simulink model "Versie1"  (Simulink 7.9)
settings: Solver=ode15s  StartTime=0.0  StopTime=10*24*3600  RelTol=1e-3
undefined symbols (not defined in the file or in its folder): B, U, x0
settings Model: Creator=psross  LastModifiedBy=M.Sparnaaij  ExtModeTrigMode=oneshot  ExtModeArmWhenConnect=off
settings DataIOCC: LimitDataPoints=off  SignalLoggingName=sigsOut
settings OptimizationCC: BooleanDataType=off
settings DebuggingCC: SaveWithParameterizedLinksMsg=none  SignalResolutionControl=TryResolveAllWithWarning  SolverPrmCheckMsg=none  MultiTaskDSMMsg=warning  MultiTaskCondExecSysMsg=none  StrictBusMsg=None
settings HardwareCC: TargetUnknown=on
settings RTWCC: IncludeERTFirstTime=on
settings GRTTargetCC: TargetFcnLib=ansi_tfl_tmw.mat  CombineOutputUpdateFcns=off  GRTInterface=on

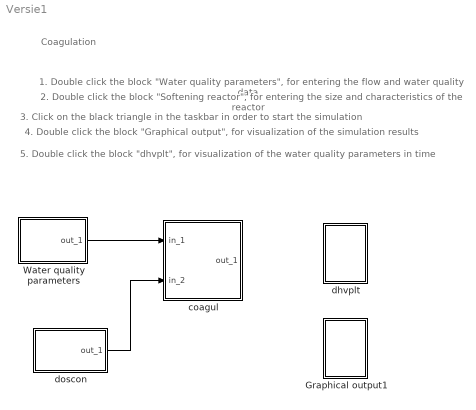
== system Versie1 ==
  note: Coagulation
  note: 3. Click on the black triangle in the taskbar in order to start the simulation
  note: 4. Double click the block "Graphical output", for visualization of the simulation results
  note: 1. Double click the block "Water quality parameters", for entering the flow and water quality data
  note: 2. Double click the block "Softening reactor", for entering the size and characteristics of the reactor
  note: 5. Double click the block "dhvplt", for visualization of the water quality parameters in time
  Graphical output1 : Subsystem
      settings: OpenFcn=coagul_g
      mask Display:
      | plot(0,0,100,100,[80,20,20],[20,20,80],[80,69,60,52,45,39,33,28,24,20],[65,65,64,61,57,52,45,37,30,20])
      | disp('');
      | text(100,100,'coagul', 'horizontalAlignment', 'right', 'verticalAlignment', 'top');
  Water quality parameters : Subsystem  Description=The water flow and the water quality data must be filled out in the 'Water quality parameters' block. Each project must start with a 'Water quality parameters' block.
      mask init:
      | filenaam='./StimelaData/rawwater.mat';
      | 
      | [Pn,Fn,Fext]=Fileprop(filenaam);
      | 
      | errstr = st_UniqName(filenaam,'filenaam=''','SubSystem','OpenFcn');
      | if errstr, error([errstr 'The filename "' filenaam '" is already in use. Choose a different filename.']), end
      | 
      | P = invruw_p(filenaam);
      | [B,x0,U]=invruw_i(filenaam);
      settings: OpenFcn=|
      | filenaam='./StimelaData/rawwater.mat';
      | st_ParameterInput('init',gcb,filenaam,'invruw');
      mask Display:
      | plot(0,0,100,100,[80 100],[ 50 50],[80 100],[ 55 55],[20 80 80 20 20],[10 10 90  90 10]);
      | disp('')
      | text(50,50,'invruw', 'horizontalAlignment', 'center', 'verticalAlignment', 'middle');
      | text(50,0,Fn, 'horizontalAlignment', 'center', 'verticalAlignment', 'base');
  coagul : Subsystem  Description=This model calculates the removal of suspended solids with a flocculation reactor.
      mask init:
      | filenaam='./StimelaData/coagulation.mat';
      | 
      | [Pn,Fn,Fext]=Fileprop(filenaam);
      | 
      | errstr = st_UniqName(filenaam,'filenaam=''','SubSystem','OpenFcn');
      | if errstr, error([errstr 'The filename "' filenaam '" is already in use. Choose a different filename.']), end
      | 
      | P = coagul_p(filenaam);
      | [B,x0,U]=coagul_i(filenaam);
      | V = st_Varia;
      settings: OpenFcn=|
      | filenaam='./StimelaData/coagulation.mat';
      | st_ParameterInput('init',gcb,filenaam,'coagul');
      mask Display:
      | plot(0,0,100,100,[80,80,20,20],[80,20,20,80],[80,20],[70,70],[50,50],[90,40],[50,61,65,67,69,70,70,69,67,65,61,50],[40,46,47,47,45,42,38,35,33,33,34,40],[50,39,35,33,31,30,30,31,33,35,39,50],[40,46,47,47,45,42,38,35,33,33,34,40])
      | disp('')
      | text(50,50,'coagul', 'horizontalAlignment', 'center', 'verticalAlignment', 'middle');
      | text(50,0,Fn, 'horizontalAlignment', 'center', 'verticalAlignment', 'base');
  dhvplt : Subsystem
      settings: OpenFcn=plotStimela2
      mask Display:
      | plot(0,0,100,100,[80,20,20],[20,20,80],[80,69,60,52,45,39,33,28,24,20],[65,65,64,61,57,52,45,37,30,20])
      | disp('');
      | text(100,100,'Stimela', 'horizontalAlignment', 'right', 'verticalAlignment', 'top');
  doscon : Subsystem  Description=doscon
      mask init:
      | filenaam='./StimelaData/doscon_p.mat';
      | 
      | [Pn,Fn,Fext]=Fileprop(filenaam);
      | 
      | errstr = st_UniqName(filenaam,'filenaam=''','SubSystem','OpenFcn');
      | if errstr, error([errstr 'The filename "' filenaam '" is already in use. Choose a different filename.']), end
      | 
      | P = doscon_p(filenaam);
      | [B,x0,U]=doscon_i(filenaam);
      settings: OpenFcn=|
      | filenaam='./StimelaData/doscon_p.mat';
      | st_ParameterInput('init',gcb,filenaam,'doscon');
      mask Display:
      | plot(0,0,100,100,[80 100],[ 50 50],[80 100],[ 55 55],[20 80 80 20 20],[10 10 90  90 10]);
      | disp('')
      | text(50,50,'doscon', 'horizontalAlignment', 'center', 'verticalAlignment', 'middle');
      | text(50,0,Fn, 'horizontalAlignment', 'center', 'verticalAlignment', 'base');
  wires:
  Water quality parameters/1(out_1) -> coagul/1(in_1)
  doscon/1(out_1) -> coagul/2(in_2)

== system Versie1/Graphical output1 ==
  note: plotten

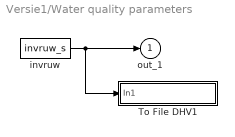
== system Versie1/Water quality parameters ==
  To File DHV1 : Subsystem  mask(To File DHV){naam=[filenaam(1:length(filenaam)-4) '_out.sti']}
      mask prompts: naam "Naam van bestand"
      mask init:
      | set_param([gcb '/To File'],'Filename',naam);
      mask Display: disp(naam)
  invruw : S-Function  FunctionName=invruw_s  Parameters=B,x0,U,P  EnableBusSupport=off
  out_1 : Outport  InitialOutput=0
  wires:
  invruw/1 -> out_1/1, To File DHV1/1(In1)

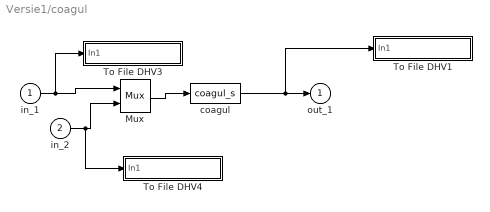
== system Versie1/coagul ==
  in_1 : Inport
  in_2 : Inport  Port=2
  Mux : Mux  Inputs=[U.Number B.Setpoints]
  To File DHV1 : Subsystem  mask(To File DHV){naam=[filenaam(1:length(filenaam)-4) '_out.sti']}
      mask prompts: naam "Naam van bestand"
      mask init:
      | set_param([gcb '/To File'],'Filename',naam);
      mask Display: disp(naam)
  To File DHV3 : Subsystem  mask(To File DHV){naam=[filenaam(1:length(filenaam)-4) '_in.sti']}
      mask prompts: naam "Naam van bestand"
      mask init:
      | set_param([gcb '/To File'],'Filename',naam);
      mask Display: disp(naam)
  To File DHV4 : Subsystem  mask(To File DHV){naam=[filenaam(1:length(filenaam)-4) '_ES.sti']}
      mask prompts: naam "Naam van bestand"
      mask init:
      | set_param([gcb '/To File'],'Filename',naam);
      mask Display: disp(naam)
  coagul : S-Function  FunctionName=coagul_s  Parameters=B,x0,U,P  EnableBusSupport=off
  out_1 : Outport  InitialOutput=0
  wires:
  in_2/1 -> To File DHV4/1(In1), Mux/2
  in_1/1 -> To File DHV3/1(In1), Mux/1
  Mux/1 -> coagul/1
  coagul/1 -> To File DHV1/1(In1), out_1/1

== system Versie1/dhvplt ==
  note: plotten

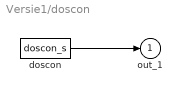
== system Versie1/doscon ==
  doscon : S-Function  FunctionName=doscon_s  Parameters=B,x0,U,P  EnableBusSupport=off
  out_1 : Outport  InitialOutput=0
  wires:
  doscon/1 -> out_1/1

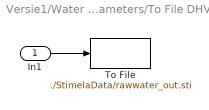
== system Versie1/Water quality parameters/To File DHV1 ==
  In1 : Inport
  To File : ToFile  Filename=./StimelaData/rawwater_out.sti  MatrixName=invruwout
  wires:
  In1/1 -> To File/1

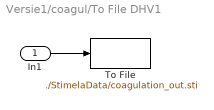
== system Versie1/coagul/To File DHV1 ==
  In1 : Inport
  To File : ToFile  Filename=./StimelaData/coagulation_out.sti  MatrixName=coagulout
  wires:
  In1/1 -> To File/1

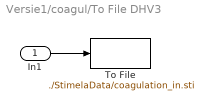
== system Versie1/coagul/To File DHV3 ==
  In1 : Inport
  To File : ToFile  Filename=./StimelaData/coagulation_in.sti  MatrixName=coagulin
  wires:
  In1/1 -> To File/1

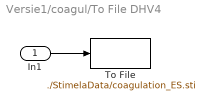
== system Versie1/coagul/To File DHV4 ==
  In1 : Inport
  To File : ToFile  Filename=./StimelaData/coagulation_ES.sti  MatrixName=coagulES
  wires:
  In1/1 -> To File/1
